simulink model "wind_turbine_10_11_21"  (R2021b)
settings: Solver=VariableStepAuto  StartTime=0.0  StopTime=10.0  RelTol=1e-3
undefined symbols (not defined in the file): id0, iq0, sigbuilder_block, w0
settings Model: Creator=Omar  LastModifiedBy=Omar

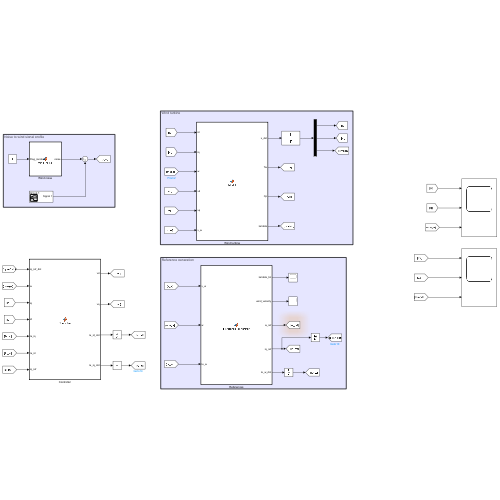
[thumbnail: Simulink's stored preview of the top-level diagram]
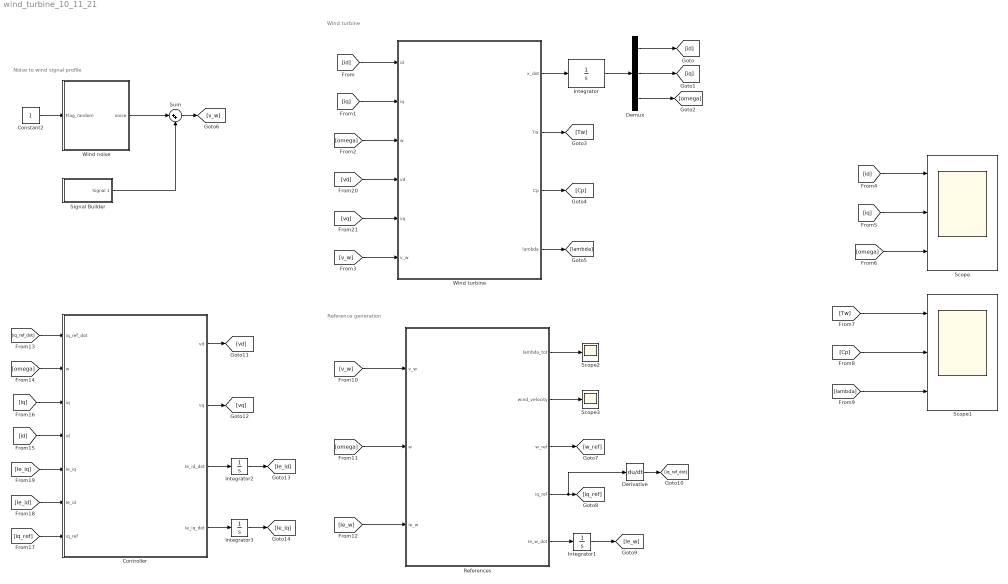
== system wind_turbine_10_11_21 ==
  note: Reference generation
  note: Noise to wind signal profile
  note: Wind turbine
  Constant2 : Constant
  Controller : MATLAB Function  TreatAsAtomicUnit=on
  Demux : Demux  Outputs=3
  Derivative : Derivative
  Integrator : Integrator  InitialCondition=[id0;iq0;w0]
  Integrator1 : Integrator
  Integrator2 : Integrator
  Integrator3 : Integrator
  References : MATLAB Function  TreatAsAtomicUnit=on
  Scope : Scope  NumInputPorts=3
  Scope1 : Scope  NumInputPorts=3
  Scope2 : Scope
  Scope3 : Scope
  Signal Builder : Subsystem  Tag=STV Subsys  LoadFcn=sigbuilder_block('load');  StartFcn=sigbuilder_block('start');  StopFcn=sigbuilder_block('stop');  ClipboardFcn=sigbuilder_block('clipboard');  mask(Sigbuilder block){tuvar=[0:10]}
      mask help: Simulink:masks:SigbuilderBlock_MD
      mask init:
      | if ~strcmp(get_param(bdroot(gcbh),'SimulationStatus'),'stopped') tuvar = sigbuilder_block('maskInit'); end
      settings: CopyFcn=sigbuilder_block('copy');  DeleteFcn=sigbuilder_block('delete');  ModelCloseFcn=sigbuilder_block('modelClose');  PreSaveFcn=sigbuilder_block('preSave');  PauseFcn=sigbuilder_block('pause');  ContinueFcn=sigbuilder_block('continue');  NameChangeFcn=sigbuilder_block('namechange');  OpenFcn=sigbuilder_block('open',[6 30 1012.5 447.75 ]);  CloseFcn=sigbuilder_block('close');
      mask Display: plot(0, 0, 100, 100,[2, 2, 32, 32, 2], [68, 8, 8, 68, 68],[32, 2], [38, 38], [32, 19, 2],[53, 60, 44], [32, 17, 17, 2],[16, 16, 31, 31]);txt = getActiveGroup(gcbh);text(2, 100, txt,'verticalAlignment', 'top');
  Sum : Sum  Inputs=|++
  Wind noise : MATLAB Function  TreatAsAtomicUnit=on
  Wind turbine : MATLAB Function  TreatAsAtomicUnit=on
  wires:
  [vd] -> Wind turbine/4(vd)
  [omega] -> Wind turbine/3(w)
  [iq] -> Wind turbine/2(iq)
  Demux/3 -> [omega]
  Demux/1 -> [id]
  Wind turbine/4(lambda) -> [lambda]
  [v_w] -> Wind turbine/6(v_w)
  Wind turbine/2(Tw) -> [Tw]
  Wind turbine/3(Cp) -> [Cp]
  [id] -> Wind turbine/1(id)
  [vq] -> Wind turbine/5(vq)
  Integrator/1 -> Demux/1
  Wind turbine/1(x_dot) -> Integrator/1
  Demux/2 -> [iq]
  Signal Builder/1(Signal 1) -> Sum/2
  Constant2/1 -> Wind noise/1(Flag_random)
  Wind noise/1(noise) -> Sum/1
  Sum/1 -> [v_w]
  [id] -> Scope/1
  [iq] -> Scope/2
  [omega] -> Scope/3
  [lambda] -> Scope1/3
  [Cp] -> Scope1/2
  [Tw] -> Scope1/1
  Derivative/1 -> [iq_ref_dot]
  [Ie_w] -> References/3(Ie_w)
  [v_w] -> References/1(v_w)
  References/2(wind_velocity) -> Scope3/1
  [omega] -> References/2(w)
  References/5(Ie_w_dot) -> Integrator1/1
  Integrator1/1 -> [Ie_w]
  References/4(iq_ref) -> Derivative/1, [iq_ref]
  References/1(lambda_tot) -> Scope2/1
  References/3(w_ref) -> [w_ref]
  [iq_ref_dot] -> Controller/1(iq_ref_dot)
  [omega] -> Controller/2(w)
  [iq] -> Controller/3(iq)
  [id] -> Controller/4(id)
  Controller/4(Ie_iq_dot) -> Integrator3/1
  Controller/3(Ie_id_dot) -> Integrator2/1
  Controller/2(vq) -> [vq]
  Controller/1(vd) -> [vd]
  Integrator2/1 -> [Ie_id]
  Integrator3/1 -> [Ie_iq]
  [iq_ref] -> Controller/7(iq_ref)
  [Ie_id] -> Controller/6(Ie_id)
  [Ie_iq] -> Controller/5(Ie_iq)

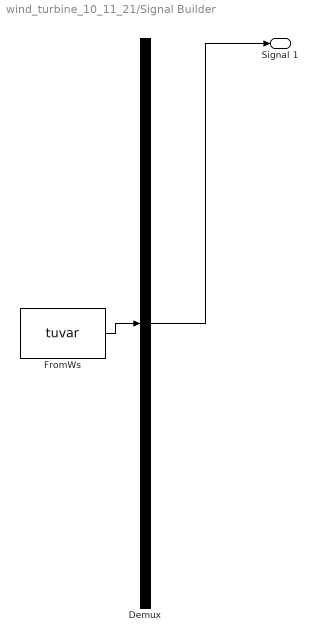
== system wind_turbine_10_11_21/Signal Builder ==
  Demux : Demux  Tag=STV Demux  Outputs=1
      settings: DisplayOption=none
  FromWs : FromWorkspace  Tag=STV FromWs  VariableName=tuvar
      SigBuilderData=|
      | common.afterFinalStr = 'Extrapolate'
      | common.sampleTime = 0
      | dataSet.timeRange = [0 10]
      | dataSet.name = 'Group 1'
      | sbobj.Groups.Name = 'Group 1'
      | sbobj.Groups.Signals.Name = 'Signal 1'
      | sbobj.Groups.Signals.XData = [0 1.9 2.9 8 8.2 10]
      | sbobj.Groups.Signals.YData = [7 7 9.4 9.4 9 9]
  Signal 1 : Outport  Tag=STV Outport
  wires:
  Demux/1 -> Signal 1/1
  FromWs/1 -> Demux/1

== matlab function wind_turbine_10_11_21/Wind noise ==
  data: Flag_random input; noise output
function noise  = wind_noise(Flag_random)%flag può essere o 0 o 1.
noise=Flag_random*0.005*randi([-10,10]);
end

== matlab function wind_turbine_10_11_21/Wind turbine ==
  data: id input; x_dot output; iq input; w input; vd input; vq input; v_w input; Tw output; Cp output; lambda output


function [x_dot,Tw,Cp,lambda] = Model(id,iq,w,vd,vq,v_w)%v_w is the wind velocity  x_dot is [id_dot; iq_dot; omega_dot]
%#eml
eml.extrinsic('evalin');%to take info from the workspace


%Loading parameters from workspace
%Inizialization

R=0;
Rs=0;
L=0;
phim=0;
p=0;
J=0;
f=0;
km=0;
c1=0;
c2=0;
c3=0;
c4=0;
c5=0;
c6=0;
rho=0;

%Take the parameters from the workspace

R=evalin('base','R');
Rs=evalin('base','Rs');
L=evalin('base','L');
phim=evalin('base','phim');
p=evalin('base','p');
J=evalin('base','J');
f=evalin('base','f');
km=evalin('base','km');
c1=evalin('base','c1');
c2=evalin('base','c2');
c3=evalin('base','c3');
c4=evalin('base','c4');
c5=evalin('base','c5');
c6=evalin('base','c6');
rho=evalin('base','rho');

%Definition of the model
lambda=(w*R)/v_w;%w is omega
C_p=c1*(c2*(1/lambda)-c3-c4)*exp(-c5*(1/lambda-c3))+c6*lambda;%has to be always greater than zero

if C_p>0
    Cp=C_p;
else
    Cp=0;
end

%real torque due to the wind
T_w=(rho*pi*R*5*Cp*w^2)/(2*lambda^3);%this too can't be less than zero T_w=kw*w^2

if T_w>0
    Tw=T_w;
else
    Tw=0;
end

%Model definition
id_dot=-(Rs/L)*id+p*w*iq+(vd/L);
iq_dot=-(Rs/L)*iq-p*w*id-(p*phim*w)/L+(vq/L);
w_dot=(km/J)*iq-(f/J)*w+(Tw/J);

x_dot=[id_dot;iq_dot;w_dot];
end

== matlab function wind_turbine_10_11_21/References ==
  data: v_w input; w input; Ie_w input; lambda_tot output; wind_velocity output; w_ref output; iq_ref output; Ie_w_dot output


function [lambda_tot,wind_velocity,w_ref,iq_ref,Ie_w_dot] = Reference_generator(v_w,w,Ie_w)%v_w is the wind velocity  x_dot is [id_dot; iq_dot; omega_dot]
%#eml
eml.extrinsic('evalin');%to take info from the workspace


%Loading parameters from workspace
%Inizialization

R=0;
Rs=0;
L=0;
phim=0;
p=0;
J=0;
f=0;
km=0;
c1=0;
c2=0;
c3=0;
c4=0;
c5=0;
c6=0;
rho=0;
lambda_max=0;

%Take the parameters from the workspace

R=evalin('base','R');
Rs=evalin('base','Rs');
L=evalin('base','L');
phim=evalin('base','phim');
p=evalin('base','p');
J=evalin('base','J');
f=evalin('base','f');
km=evalin('base','km');
c1=evalin('base','c1');
c2=evalin('base','c2');
c3=evalin('base','c3');
c4=evalin('base','c4');
c5=evalin('base','c5');
c6=evalin('base','c6');
rho=evalin('base','rho');
lambda_max=evalin('base','lambda_max');

%Real tip speed ratio
lambda=(w*R)/v_w;

C_p=c1*(c2*(1/lambda)-c3-c4)*exp(-c5*(1/lambda-c3))+c6*lambda;%has to be always greater than zero


if C_p>0
    Cp=C_p;
else
    Cp=0;
end

%real torque due to the wind
kw=(rho*pi*R*5*Cp*w^2)/(2*lambda^3);%this too can't be less than zero T_w=kw*w^2
T_w=kw*w^2;
if T_w>0
    Tw=T_w;
else
    Tw=0;
end

%estimation of the wind velocity

v_wh0=7.5;%Initial value of the estimated wind velocity
lambda_h=(w*R)/v_wh0;%Initial value of the estimated tip speed ratio
C_ph=c1*(c2*(1/lambda_h)-c3-c4)*exp(-c5*(1/lambda_h-c3))+c6*lambda_h;

if C_ph>0
    Cph=C_ph;
else
    Cph=0;
end

kw0=(rho*pi*R*5*Cph*w^2)/(2*lambda_h^3);%this too can't be less than zero T_w=kw*w^2
T_w0=kw0*w^2;
if T_w0>0
    Tw0=T_w0;
else
    Tw0=0;
end

%Now I start with the estimation

%derivative of Cp
a1=c1*(-c2*c3/lambda_h-c2*(-c3*lambda_h+1)/lambda_h^2)*exp(-c5*(-c3*lambda_h+1)/lambda_h+c4)+c1*(c2*(-c3*lambda_h+1)/lambda_h-c4)*(c5*c3/lambda_h+c5*(-c3*lambda_h+1)/lambda_h^2)*exp(-c5*(-c3*lambda_h+1)/lambda_h+c4)+c6;
a2=3*(c1*(c2*(-c3*lambda_h+1)/lambda_h-c4)*exp(-c5*(-c3*lambda_h+1)/lambda_h+c4)+c6*lambda_h);
DCp=a1/lambda_h^3-a2/lambda_h^4;

%Measured power
Pm=kw*w^3;

f_lambda=Pm-kw0*w^3;%this is were I want to apply the Newt Raph method
df_lambda=-(rho*pi*R^5*w^3*DCp)/2;

%Now NR method
N=109;%if I increase or reduce it does not approximate as well it's a sensitive parameter
%this number sinchronizes the ode45 simulink with the nr method

for i=1:N
    lambda_h=lambda_h-f_lambda/df_lambda;
end

%I compute again C_ph and T_w0 that uses lambda_h obtained with NR method
C_ph=c1*(c2*(1/lambda_h)-c3-c4)*exp(-c5*(1/lambda_h-c3))+c6*lambda_h;

if C_ph>0
    Cph=C_ph;
else
    Cph=0;
end

kw0=(rho*pi*R*5*Cph*w^2)/(2*lambda_h^3);%this too can't be less than zero T_w=kw*w^2
T_w0=kw0*w^2;
if T_w0>0
    Tw0=T_w0;
else
    Tw0=0;
end

lambda_tot=[lambda;lambda_h];
v_wh=w*R/lambda_h;
wind_velocity=[v_w;v_wh];

w_ref=lambda_max*v_wh/R;

kp2=30;
ki2=2*kp2;

e_w=w-w_ref;
Ie_w_dot=e_w;
iq_ref=J/km*(-(f/J)*w+(Tw0/J)+kp2*e_w+ki2*Ie_w);

end

== matlab function wind_turbine_10_11_21/Controller ==
  data: iq_ref_dot input; vd output; vq output; w input; iq input; id input; Ie_iq input; Ie_id input; iq_ref input; Ie_id_dot output; Ie_iq_dot output


function[vd,vq,Ie_id_dot,Ie_iq_dot] = Controller(iq_ref_dot,w,iq,id,Ie_iq,Ie_id,iq_ref)%v_w is the wind velocity  x_dot is [id_dot; iq_dot; omega_dot]
%#eml
eml.extrinsic('evalin');%to take info from the workspace


%Loading parameters from workspace
%Inizialization

R=0;
Rs=0;
L=0;
phim=0;
p=0;
J=0;
f=0;
km=0;
c1=0;
c2=0;
c3=0;
c4=0;
c5=0;
c6=0;
rho=0;
lambda_max=0;

%Take the parameters from the workspace

R=evalin('base','R');
Rs=evalin('base','Rs');
L=evalin('base','L');
phim=evalin('base','phim');
p=evalin('base','p');
J=evalin('base','J');
f=evalin('base','f');
km=evalin('base','km');
c1=evalin('base','c1');
c2=evalin('base','c2');
c3=evalin('base','c3');
c4=evalin('base','c4');
c5=evalin('base','c5');
c6=evalin('base','c6');
rho=evalin('base','rho');
lambda_max=evalin('base','lambda_max');

%Definition of the controller

id_ref=0;%best choice is putting this to zero
e_id=id-id_ref;
Ie_id_dot=e_id;

kp1=30;
ki1=2*kp1;

vd=L*((Rs/L)*id-p*w*iq-kp1*e_id-ki1*Ie_id);

e_iq=iq-iq_ref;
Ie_iq_dot=e_iq;

kp3=30;
ki3=2*kp3;

vq=L*((Rs/L)*iq+p*w*id+(p*phim*w)/L-kp3*e_iq-ki3*Ie_iq+iq_ref_dot);
end
